simulink model "ldpc_dvbs2_model"  (R2020b)
settings: Solver=FixedStepDiscrete  StartTime=0.0  StopTime=360*135  RelTol=1e-3
libraries: hdlsllib x3, simulink x2
settings Model: DataTypeOverride=Off  Creator=wardo  LastModifiedBy=wardo
settings DataIOCC: LimitDataPoints=on  SaveOutput=off  SaveTime=off
settings OptimizationCC: BlockReduction=off  ConditionallyExecuteInputs=off  DefaultParameterBehavior=Inlined  LifeSpan=inf
settings DebuggingCC: AlgebraicLoopMsg=error  SingleTaskRateTransMsg=error  AllowSymbolicDim=off  StrictBusMsg=ErrorOnBusTreatedAsVector  SFUnexpectedBacktrackingDiag=warning  SFNoUnconditionalDefaultTransitionDiag=warning  SFExecutionAtInitializationDiag=none  ArithmeticOperatorsInVariantConditions=warning
settings HardwareCC: ProdBitPerPointer=32  ProdBitPerSizeT=32  ProdBitPerPtrDiffT=32  ProdLargestAtomicFloat=None  ProdIntDivRoundTo=Undefined  ProdEndianess=Unspecified  ProdWordSize=32  ProdHWDeviceType=ASIC/FPGA->ASIC/FPGA  ProdEqTarget=off
settings SFSimCC: SimUseLocalCustomCode=off  CustomCodeUndefinedFunction=UseInterfaceOnly
settings RTWCC: RTWUseLocalCustomCode=off
settings CodeAppCC: StateflowObjectComments=on
settings GRTTargetCC: TargetLangStandard=C89/C90 (ANSI)
settings ConfigComp: CovScope=ReferencedModels  CovMetricSettings=dw  CovSaveCumulativeToWorkspaceVar=on  CovSaveSingleToWorkspaceVar=on  CovExternalEMLEnable=off  CovSFcnEnable=off

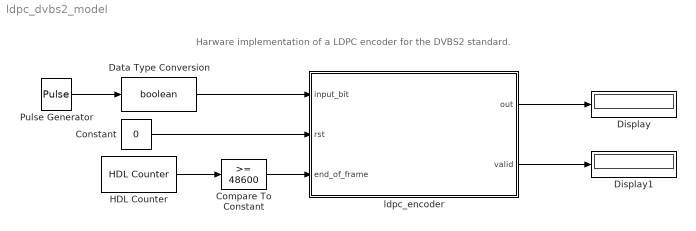
== system ldpc_dvbs2_model ==
  note: Harware implementation of a LDPC encoder for the DVBS2 standard.
  Compare To Constant : simulink/Logic and Bit Operations/Compare To Constant  relop=>=  const=48600  OutDataTypeStr=boolean
  Constant : Constant  Value=0  OutDataTypeStr=boolean
  Data Type Conversion : DataTypeConversion  OutDataTypeStr=boolean
  Display : Display
  Display1 : Display
  HDL Counter : hdlsllib/Sources/HDL Counter  CountType=Count limited  CountInit=1  CountStep=1  CountMax=48600  CountFromType=Initial value  CountFrom=1  CountResetPort=off  CountLoadPort=off  CountEnbPort=off  CountDirPort=off  CountDataType=Unsigned  CountWordLen=16  CountFracLen=0  CountSampTime=1
  Pulse Generator : DiscretePulseGenerator  PulseType=Time based  PulseWidth=50
  ldpc_encoder : Subsystem
  wires:
  ldpc_encoder/1(out) -> Display/1
  Constant/1 -> ldpc_encoder/2(rst)
  Pulse Generator/1 -> Data Type Conversion/1
  Data Type Conversion/1 -> ldpc_encoder/1(input_bit)
  Compare To Constant/1 -> ldpc_encoder/3(end_of_frame)
  HDL Counter/1 -> Compare To Constant/1
  ldpc_encoder/2(valid) -> Display1/1

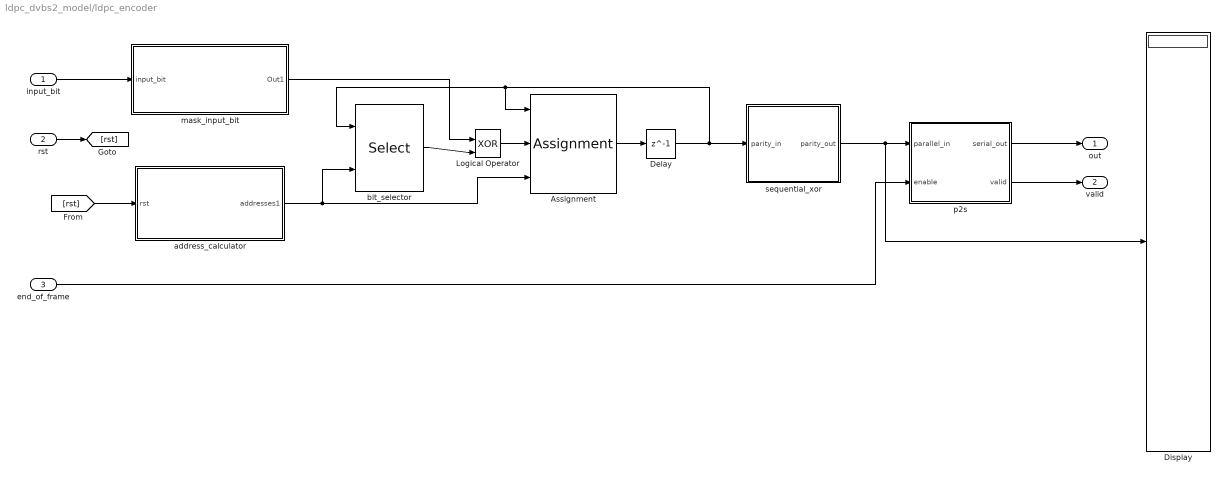
== system ldpc_dvbs2_model/ldpc_encoder ==
  input_bit : Inport
  rst : Inport  Port=2
  end_of_frame : Inport  Port=3
  Assignment : Assignment  IndexMode=Zero-based  IndexOptions=Index vector (port)  Indices=1  OutputSizes=1
  Delay : Delay  DelayLength=1  InitialCondition=[zeros(16200, 1); 1]
  Display : Display
  Logical Operator : Logic  Operator=XOR  IconShape=distinctive  AllPortsSameDT=off  OutDataTypeStr=fixdt(0,1)
  address_calculator : Subsystem
  bit_selector : Selector  IndexMode=Zero-based  InputPortWidth=16201  IndexOptions=Index vector (port)  Indices=[1 3]  OutputSizes=1
  mask_input_bit : Subsystem
  p2s : MATLAB Function  TreatAsAtomicUnit=on  mask{input_length=16200}
  sequential_xor : MATLAB Function  TreatAsAtomicUnit=on  mask{num_parity_bits=16200}
  out : Outport  VectorParamsAs1DForOutWhenUnconnected=off
  valid : Outport  Port=2  VectorParamsAs1DForOutWhenUnconnected=off
  wires:
  bit_selector/1 -> Logical Operator/2
  Logical Operator/1 -> Assignment/2
  mask_input_bit/1(Out1) -> Logical Operator/1
  input_bit/1 -> mask_input_bit/1(input_bit)
  rst/1 -> [rst]
  Assignment/1 -> Delay/1
  Delay/1 -> Assignment/1, bit_selector/1, sequential_xor/1(parity_in)
  address_calculator/1(addresses1) -> Assignment/3, bit_selector/2
  [rst] -> address_calculator/1(rst)
  sequential_xor/1(parity_out) -> Display/1, p2s/1(parallel_in)
  p2s/1(serial_out) -> out/1
  end_of_frame/1 -> p2s/2(enable)
  p2s/2(valid) -> valid/1

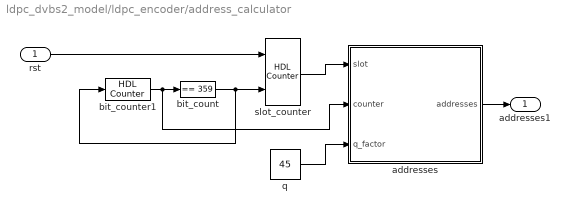
== system ldpc_dvbs2_model/ldpc_encoder/address_calculator ==
  rst : Inport
  addresses : MATLAB Function  TreatAsAtomicUnit=on  mask{bit_addresses=uint16([[0 6385 7901 14611 13389 11200 3252 5243 2504 2722 821 7374]; [1 11359 2698 357 13824 12772 7244 6752 15310 852 2001 11417]; [2 7862 7977 6321 13612 12197 14449 15137 13860 1708 6399 13444]; [3 1560 11804 6975 13292 3646 3812 8772 7306 5795 14327 7866]; [4 7626 11407 14599 9689 1628 2113 10809 9283 1230 15241 4870]; [5 1610 5699 15876 9446 12515 1400 6303 5411 14181 13925 7358]; [6 4059 8836 3405 7853 7992 15336 5970 10368 10278 9675 4651]; [7 4441 3963 9153 2109 12683 7459 12030 12221 629 15212 406]; [8 6007 8411 5771 3497 543 14202 875 9186 6235 13908 3563]; [9 3232 6625 4795 546 9781 2071 7312 3399 7250 4932 12652]; [10 8820 10088 11090 7069 6585 13134 10158 7183 488 7455 9238]; [11 1903 10818 119 215 7558 11046 10615 11545 14784 7961 15619]; [12 3655 8736 4917 15874 5129 2134 15944 14768 7150 2692 1469]; [13 8316 3820 505 8923 6757 806 7957 4216 15589 13244 2622]; [14 14463 4852 15733 3041 11193 12860 13673 8152 6551 15108 8758]; [15 3149 11981 16200 16200 16200 16200 16200 16200 16200 16200 16200]; [16 13416 6906 16200 16200 16200 16200 16200 16200 16200 16200 16200]; [17 13098 13352 16200 16200 16200 16200 16200 16200 16200 16200 16200]; [18 2009 14460 16200 16200 16200 16200 16200 16200 16200 16200 16200]; [19 7207 4314 16200 16200 16200 16200 16200 16200 16200 16200 16200]; [20 3312 3945 16200 16200 16200 16200 16200 16200 16200 16200 16200]; [21 4418 6248 16200 16200 16200 16200 16200 16200 16200 16200 16200]; [22 2669 13975 16200 16200 16200 16200 16200 16200 16200 16200 16200]; [23 7571 9023 16200 16200 16200 16200 16200 16200 16200 16200 16200]; [24 14172 2967 16200 16200 16200 16200 16200 16200 16200 16200 16200]; [25 7271 7138 16200 16200 16200 16200 16200 16200 16200 16200 16200]; [26 6135 13670 16200 16200 16200 16200 16200 16200 16200 16200 16200]; [27 7490 14559 16200 16200 16200 16200 16200 16200 16200 16200 16200]; [28 8657 2466 16200 16200 16200 16200 16200 16200 16200 16200 16200]; [29 8599 12834 16200 16200 16200 16200 16200 16200 16200 16200 16200]; [30 3470 3152 16200 16200 16200 16200 16200 16200 16200 16200 16200]; [31 13917 4365 16200 16200 16200 16200 16200 16200 16200 16200 16200]; [32 6024 13730 16200 16200 16200 16200 16200 16200 16200 16200 16200]; [33 10973 14182 16200 16200 16200 16200 16200 16200 16200 16200 16200]; [34 2464 13167 16200 16200 16200 16200 16200 16200 16200 16200 16200]; [35 5281 15049 16200 16200 16200 16200 16200 16200 16200 16200 16200]; [36 1103 1849 16200 16200 16200 16200 16200 16200 16200 16200 16200]; [37 2058 1069 16200 16200 16200 16200 16200 16200 16200 16200 16200]; [38 9654 6095 16200 16200 16200 16200 16200 16200 16200 16200 16200]; [39 14311 7667 16200 16200 16200 16200 16200 16200 16200 16200 16200]; [40 15617 8146 16200 16200 16200 16200 16200 16200 16200 16200 16200]; [41 4588 11218 16200 16200 16200 16200 16200 16200 16200 16200 16200]; [42 13660 6243 16200 16200 16200 16200 16200 16200 16200 16200 16200]; [43 8578 7874 16200 16200 16200 16200 16200 16200 16200 16200 16200]; [44 11741 2686 16200 16200 16200 16200 16200 16200 16200 16200 16200]; [0 1022 1264 16200 16200 16200 16200 16200 16200 16200 16200 16200]; [1 12604 9965 16200 16200 16200 16200 16200 16200 16200 16200 16200]; [2 8217 2707 16200 16200 16200 16200 16200 16200 16200 16200 16200]; [3 3156 11793 16200 16200 16200 16200 16200 16200 16200 16200 16200]; [4 354 1514 16200 16200 16200 16200 16200 16200 16200 16200 16200]; [5 6978 14058 16200 16200 16200 16200 16200 16200 16200 16200 16200]; [6 7922 16079 16200 16200 16200 16200 16200 16200 16200 16200 16200]; [7 15087 12138 16200 16200 16200 16200 16200 16200 16200 16200 16200]; [8 5053 6470 16200 16200 16200 16200 16200 16200 16200 16200 16200]; [9 12687 14932 16200 16200 16200 16200 16200 16200 16200 16200 16200]; [10 15458 1763 16200 16200 16200 16200 16200 16200 16200 16200 16200]; [11 8121 1721 16200 16200 16200 16200 16200 16200 16200 16200 16200]; [12 12431 549 16200 16200 16200 16200 16200 16200 16200 16200 16200]; [13 4129 7091 16200 ...(+5412 chars)]]);, num_parity_bits=16200}
  bit_count : simulink/Logic and Bit Operations/Compare To Constant  relop===  const=359  OutDataTypeStr=boolean
  bit_counter1 : hdlsllib/Sources/HDL Counter  CountType=Count limited  CountInit=0  CountStep=1  CountMax=359  CountFromType=Initial value  CountFrom=0  CountResetPort=on  CountLoadPort=off  CountEnbPort=off  CountDirPort=off  CountDataType=Unsigned  CountWordLen=9  CountFracLen=0  CountSampTime=1
  q : Constant  Value=45  OutDataTypeStr=uint8  SampleTime=-1
  slot_counter : hdlsllib/Sources/HDL Counter  CountType=Count limited  CountInit=1  CountStep=1  CountMax=135  CountFromType=Initial value  CountFrom=1  CountResetPort=on  CountLoadPort=off  CountEnbPort=on  CountDirPort=off  CountDataType=Unsigned  CountWordLen=8  CountFracLen=0  CountSampTime=1
  addresses1 : Outport
  wires:
  addresses/1(addresses) -> addresses1/1
  bit_counter1/1 -> addresses/2(counter), bit_count/1
  bit_count/1 -> bit_counter1/1, slot_counter/2
  q/1 -> addresses/3(q_factor)
  rst/1 -> slot_counter/1
  slot_counter/1 -> addresses/1(slot)

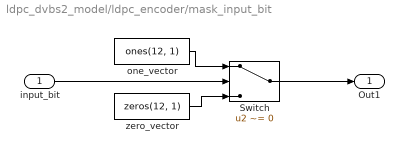
== system ldpc_dvbs2_model/ldpc_encoder/mask_input_bit ==
  input_bit : Inport
  Switch : Switch  Criteria=u2 ~= 0
  one_vector : Constant  Value=ones(12, 1)  OutDataTypeStr=fixdt(0,1,0)  SampleTime=-1
  zero_vector : Constant  Value=zeros(12, 1)  OutDataTypeStr=fixdt(0,1,0)  SampleTime=-1
  Out1 : Outport
  wires:
  zero_vector/1 -> Switch/3
  input_bit/1 -> Switch/2
  Switch/1 -> Out1/1
  one_vector/1 -> Switch/1

== matlab function ldpc_dvbs2_model/ldpc_encoder/sequential_xor ==
  settings: fimath=fimath('RoundingMethod', 'Floor','OverflowAction', 'Wrap','ProductMode', 'FullPrecision', 'SumMode', 'FullPrecision')
  data: parity_in input; parity_out output; num_parity_bits parameter uint16
function parity_out = sequential_xor(parity_in, num_parity_bits)
%#codegen
parity_out = fi(zeros(num_parity_bits, 1), 0, 1, 0);
parity_out(1) = parity_in(1);
for i = 2:num_parity_bits
    parity_out(i) = xor(parity_in(i), parity_out(i-1));
end

== matlab function ldpc_dvbs2_model/ldpc_encoder/address_calculator/addresses ==
  settings: fimath=fimath('RoundingMethod', 'Floor','OverflowAction', 'Wrap','ProductMode', 'FullPrecision', 'SumMode', 'FullPrecision')
  data: slot input; counter input; q_factor input; addresses output uint16; bit_addresses parameter uint16; num_parity_bits parameter uint16
function addresses = address_generator(slot, counter, q_factor, bit_addresses, num_parity_bits)
%#codegen
buffer = uint16(bit_addresses(slot, :) + counter*q_factor);
addresses = buffer - uint16(num_parity_bits) .* uint16(buffer >= num_parity_bits);

== matlab function ldpc_dvbs2_model/ldpc_encoder/p2s ==
  settings: fimath=fimath('RoundingMethod', 'Floor','OverflowAction', 'Wrap','ProductMode', 'FullPrecision', 'SumMode', 'FullPrecision')
  data: parallel_in input; serial_out output fixdt(0,1,0); enable input; input_length parameter uint16; valid output
function [serial_out, valid] = p2s_buffer(parallel_in, enable, input_length)
%#codegen

state_iddle = 0;
state_reading = 1;

persistent moore_state_machine;
if isempty(moore_state_machine)
    moore_state_machine = 0;
end

persistent counter;
if isempty(counter)
    counter = fi(1, 0, 16, 0);
end

persistent buffer;
if isempty(buffer)
    buffer = parallel_in;
end

switch moore_state_machine
    case state_iddle
        serial_out = fi(0, 0, 1, 0);
        valid      = fi(0, 0, 1, 0);
        if enable
            moore_state_machine = state_reading;
            serial_out          = buffer(counter);
            counter             = fi(counter + 1, 0, 16, 0);
        end
    case state_reading
        serial_out = buffer(counter);
        counter    = fi(counter + 1, 0, 16, 0);
        valid      = fi(1, 0, 1, 0);
        if(counter > input_length)
            moore_state_machine = state_iddle;
        end
    otherwise
        serial_out = fi(0, 0, 1, 0);
        valid      = fi(0, 0, 1, 0);
end
